simulink model "Siddarth_Kachu_FinalProject_Model"  (R2025a)
settings: Solver=FixedStepDiscrete  StartTime=0.0  StopTime=0.5  FixedStep=1e-6  RelTol=1e-3
model workspace (MAT data in the model file):
  AngularVelocity = Simulink.Parameter
  AngularVelocity.Value = 209.439510239
  AngularVelocity.Complexity = 'real'
  AngularVelocity.Dimensions = [1 1]
  AngularVelocity.DataType = 'auto'
  CounterTs = Simulink.Parameter
  CounterTs.Value = 20
  CounterTs.Complexity = 'real'
  CounterTs.Dimensions = [1 1]
  CounterTs.DataType = 'auto'
  Current_ZeroThreshold = Simulink.Parameter
  Current_ZeroThreshold.Value = 2.5
  Current_ZeroThreshold.Complexity = 'real'
  Current_ZeroThreshold.Dimensions = [1 1]
  Current_ZeroThreshold.DataType = 'auto'
  Nrpm = 2000
  OutputVoltages = [-5 -4 -3 -2 -1 0 1 2 3 4 5]
  RotorPoles = 8
  Rph = Simulink.Parameter
  Rph.Value = 0.4
  Rph.Complexity = 'real'
  Rph.Dimensions = [1 1]
  Rph.DataType = 'auto'
  Ts = Simulink.Parameter
  Ts.Value = 1e-06
  Ts.Complexity = 'real'
  Ts.Dimensions = [1 1]
  Ts.DataType = 'auto'
  Vdc = Simulink.Parameter
  Vdc.Value = 300
  Vdc.Complexity = 'real'
  Vdc.Dimensions = [1 1]
  Vdc.DataType = 'auto'
values from neighbouring files (symbols this model uses):
  elecAngleArray = [0 1.0000032 2.0000064 3.0000096 4.0000128 5.000016 6.0000192 7.0000224 8.0000256 9.0000288 10.000032 11.0000352 ... (360 elements, 360x1)]    [MPC_Controller_Final_Workspace.mat]
  LUT_currentMatrix = zeros(N_angles,N_fluxlink)    [Final_Project_Script.m]    (also in MPC_Controller_Final_Workspace.mat = [0 0 0 0 0 0 0 0 0 0 0 0 ... (129600 elements, 360x360)])
  targetArray = linspace(min(fluxLinkageMatrix(:)),max(fluxLinkageMatrix(:)),N_fluxlink)    [Final_Project_Script.m]    (also in MPC_Controller_Final_Workspace.mat = [0 0.00022373205571 0.000447464111421 0.000671196167131 0.00)
libraries: spsDiodeLib x12, spsIGBTDiodeLib x12, simulink x6, spsControlledCurrentSourceLib x3, spsVoltageMeasurementLib x3, spsDCVoltageSourceLib x2, simulink_need_slupdate x2, sps_lib x1
settings Model: Creator=kachus1  LastModifiedBy=kachus1
settings DataIOCC: ReturnWorkspaceOutputs=off

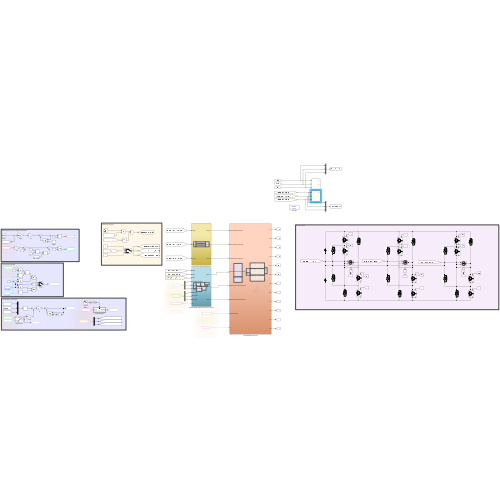
[thumbnail: Simulink's stored preview of the top-level diagram]
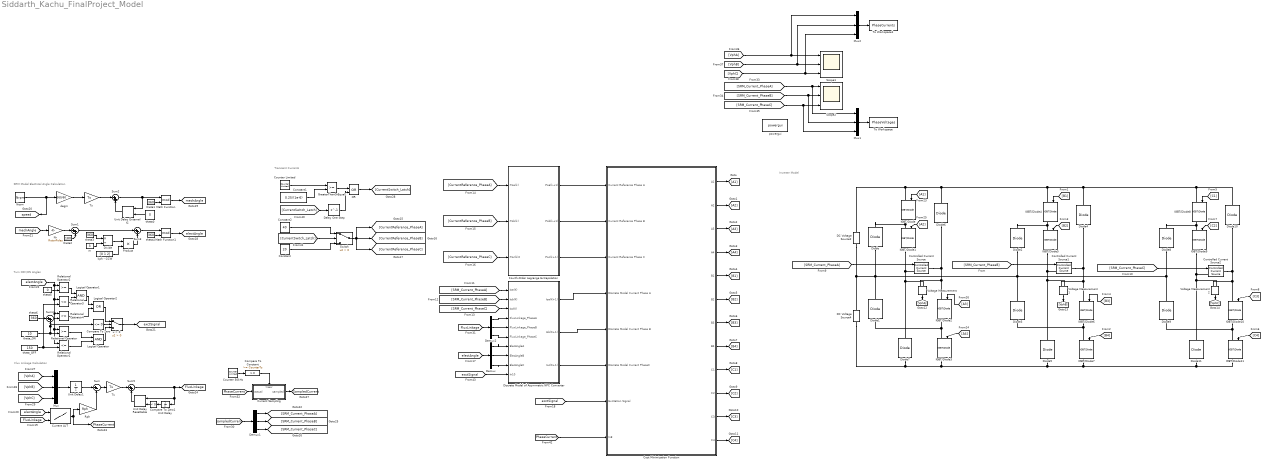
== system Siddarth_Kachu_FinalProject_Model ==
  note: Inverter Model
  note: Transient Currents
  note: Flux Linkage Calculation
  note: Turn OFF/ON Angles
  note: SRM Model Electrical Angle Calculation
  Compare To Constant : simulink/Logic and Bit Operations/Compare To Constant  relop=>=  const=CounterTs  OutDataTypeStr=boolean
  Compare To Zero : simulink/Logic and Bit Operations/Compare To Zero  relop=<=  OutDataTypeStr=boolean
  Compare To Zero1 : simulink/Logic and Bit Operations/Compare To Zero  relop=<  OutDataTypeStr=boolean
  Constant : Constant  Value=20
  Constant1 : Constant  Value=0.25/(1e-6)
  Constant2 : Constant  Value=40
  Controlled Current Source : spsControlledCurrentSourceLib/Controlled Current Source  Initialize=on  Source_Type=DC  Amplitude=0  Phase=0  Frequency=0  Measurements=None
  Controlled Current Source1 : spsControlledCurrentSourceLib/Controlled Current Source  Initialize=on  Source_Type=DC  Amplitude=0  Phase=0  Frequency=0  Measurements=None
  Controlled Current Source2 : spsControlledCurrentSourceLib/Controlled Current Source  Initialize=on  Source_Type=DC  Amplitude=0  Phase=0  Frequency=0  Measurements=None
  Cost Minimization Function : Subsystem
  Counter 50kHz : simulink/Sources/Counter Limited  uplimit=CounterTs  tsamp=-1
  Counter Limited : simulink/Sources/Counter Limited  uplimit=0.25/(1e-6)  tsamp=-1
  Current LUT : Lookup_n-D  BreakpointsForDimension1=elecAngleArray  BreakpointsForDimension2=targetArray  Table=LUT_currentMatrix  InternalRulePriority=Speed  RndMeth=Simplest
      settings: InputPortMap=u0,u1
  Current Sampling : Subsystem  TreatAsAtomicUnit=on
  DC Voltage Source2 : spsDCVoltageSourceLib/DC Voltage Source  Amplitude=150  Measurements=None
  DC Voltage Source4 : spsDCVoltageSourceLib/DC Voltage Source  Amplitude=150  Measurements=None
  Delay One Step : Delay  DelayLength=1
  Demux : Demux  Outputs=3
  Demux1 : Demux  Outputs=3
  Demux2 : Demux  Outputs=3
  Diode{,1..11} (12 alike) : spsDiodeLib/Diode  Ron=0.001  Lon=0  Vf=0  IC=0  UseSnubber=0  Rs=500  Cs=250e-9  Measurements=off
  Discrete Model of Asymmetric NPC Converter : Subsystem
  Divide : Product  Inputs=*/
  Fourth-Order Lagrange Extrapolation : Subsystem
  GreaterThanOrEqual : RelationalOperator  OutDataTypeStr=boolean  RndMeth=Simplest  InputSameDT=off
  IGBT/Diode{,1..11} (12 alike) : spsIGBTDiodeLib/IGBT//Diode  Ron=1e-3  Rs=1e5  Cs=inf  Measurements=on
  Logical Operator : Logic  AllPortsSameDT=off  OutDataTypeStr=boolean
  Logical Operator1 : Logic  AllPortsSameDT=off  OutDataTypeStr=boolean
  Logical Operator2 : Logic  Operator=OR  AllPortsSameDT=off  OutDataTypeStr=boolean
  Math Function : Math  Operator=mod  SignedPower=on
  Math Function1 : Math  Operator=mod  SignedPower=on
  Mux : Mux  Inputs=3
  Mux1 : Mux  Inputs=3
  Mux2 : Mux  Inputs=3
  Nr : Gain  Gain=RotorPoles
  Nrpm : Constant  Value=Nrpm
  OR : Logic  Operator=OR  IconShape=distinctive  AllPortsSameDT=off  OutDataTypeStr=boolean
  Product : Product
  Relational Operator : RelationalOperator  OutDataTypeStr=boolean  InputSameDT=off
  Relational Operator1 : RelationalOperator  Operator=<=  OutDataTypeStr=boolean  InputSameDT=off
  Relational Operator2 : RelationalOperator  OutDataTypeStr=boolean  InputSameDT=off
  Relational Operator3 : RelationalOperator  Operator=<=  OutDataTypeStr=boolean  InputSameDT=off
  Relational Operator4 : RelationalOperator  OutDataTypeStr=boolean  InputSameDT=off
  Rph : Gain  Gain=Rph
  Scope1 : Scope  NumInputPorts=3
      settings: ActiveDisplayYMinimum=-375.09564073144674  ActiveDisplayYMaximum=375.01062674793855
  Scope2 : Scope  NumInputPorts=3
      settings: ActiveDisplayYMinimum=-5.5949717067570885  ActiveDisplayYMaximum=48.44572805476993
  Sum : Sum  Inputs=|+-
  Sum{1..5} (5 alike) : Sum  Inputs=|++
  Switch : Switch  Criteria=u2 > Threshold  SaturateOnIntegerOverflow=off  InputSameDT=off
  To Workspace : ToWorkspace  VariableName=PhaseVoltages  SaveFormat=Structure With Time  SampleTime=-1
  To Workspace1 : ToWorkspace  VariableName=PhaseCurrents  SaveFormat=Structure With Time  SampleTime=-1
  Ts : Gain  Gain=Ts
  "Ts " : Gain  Gain=Ts
  Unit Delay : UnitDelay  SampleTime=-1  HasFrameUpgradeWarning=on
  Unit Delay External IC : simulink_need_slupdate/Unit Delay External IC  tsamp=-1
  Unit Delay Resettable : simulink_need_slupdate/Unit Delay Resettable  vinit=0.0  tsamp=-1
  Unit Delay1 : UnitDelay  SampleTime=-1  HasFrameUpgradeWarning=on
  Voltage Measurement : spsVoltageMeasurementLib/Voltage Measurement  PhasorSimulation=off  OutputType=Complex  PSBequivalent=0
  Voltage Measurement1 : spsVoltageMeasurementLib/Voltage Measurement  PhasorSimulation=off  OutputType=Complex  PSBequivalent=0
  Voltage Measurement2 : spsVoltageMeasurementLib/Voltage Measurement  PhasorSimulation=off  OutputType=Complex  PSBequivalent=0
  deg/s : Gain  Gain=360/60
  kph - CCW : Constant  Value=[0 1 2]
  m : Constant  Value=3
  powergui : sps_lib/powergui  Priority=1  SimulationMode=Discrete  SampleTime=1e-6  frequency=60  Iterations=50  frequencyindice=0  Pbase=100e6  ErrMax=1e-4  UnitsV=kV  UnitsW=MW  buscounter=0  FunctionMessages=off  echomessages=off  EnableUseOfTLC=off  CurrentSourceSwitches=off  DisableSnubberDevices=off  DisableRonSwitches=off  DisableVfSwitches=off  DisplayEquations=off  AutomaticDiscreteSolvers=off  SolverType=Tustin/Backward Euler (TBE)  Interpol=off  ExternalGateDelay=off  methode=off  Ts=100  x0status=blocks  SPID=on  SwTol=0  HookPort=off  NonlinearTolerance=1e-4  nMaxIteration=100  ContinueOnMaxIteration=off  RestoreLinks=warning  ResistiveCurrentMeasurement=off  Frange=[0:2:500]  Ylog=off  Xlog=on  ShowGrid=off  save=off  variable=ZData  structure=0  ZoomFFT=off  StartTime=0.0  cycles=1  DisplayStyle=1  fundamental=60  FreqAxis=off  MaxFrequency=1000  frequencyindicesteady=1  RmsSteady=1  display=off
  theta0 : Constant  Value=0
  theta{1,3..4,6} (4 alike) : Constant  Value=360
  theta2 : Constant  Value=180
  theta5 : Constant  Value=0
  theta_OFF : Constant  Value=150
  theta_ON : Constant  Value=10
  u > 0 : Switch  Criteria=u2 > Threshold  SaturateOnIntegerOverflow=off  InputSameDT=off
  tag scope: FluxLinkage=global, PhaseCurrent=global, SampledCurrent=global, electAngle=global, exctSignal=global, mechAngle=global, speed=global
  wires:
  [A2] -> IGBT/Diode1/1
  [A1] -> IGBT/Diode/1
  [A3] -> IGBT/Diode2/1
  [A4] -> IGBT/Diode3/1
  [B1] -> IGBT/Diode4/1
  [B2] -> IGBT/Diode5/1
  [B3] -> IGBT/Diode6/1
  [B4] -> IGBT/Diode7/1
  [C3] -> IGBT/Diode10/1
  [C4] -> IGBT/Diode11/1
  [C2] -> IGBT/Diode9/1
  [C1] -> IGBT/Diode8/1
  [SRM_Current_PhaseB] -> Controlled Current Source1/1
  [SRM_Current_PhaseA] -> Controlled Current Source/1
  [SRM_Current_PhaseC] -> Controlled Current Source2/1
  Cost Minimization Function/1(A1) -> [A1]
  Cost Minimization Function/2(A2) -> [A2]
  Cost Minimization Function/3(A3) -> [A3]
  Cost Minimization Function/4(A4) -> [A4]
  Cost Minimization Function/5(B1) -> [B1]
  Cost Minimization Function/6(B2) -> [B2]
  Cost Minimization Function/7(B3) -> [B3]
  Cost Minimization Function/8(B4) -> [B4]
  Cost Minimization Function/11(C3) -> [C3]
  Cost Minimization Function/10(C2) -> [C2]
  Cost Minimization Function/9(C1) -> [C1]
  Cost Minimization Function/12(C4) -> [C4]
  Discrete Model of Asymmetric NPC Converter/1(Ioa(K+1)) -> Cost Minimization Function/4(Discrete Model Current Phase A)
  Fourth-Order Lagrange Extrapolation/1(I*oa(k+1)) -> Cost Minimization Function/1(Current Reference Phase A)
  Fourth-Order Lagrange Extrapolation/2(I*ob(k+1)) -> Cost Minimization Function/2(Current Reference Phase B)
  Fourth-Order Lagrange Extrapolation/3(I*oc(k+1)) -> Cost Minimization Function/3(Current Reference Phase C)
  [SRM_Current_PhaseA] -> Discrete Model of Asymmetric NPC Converter/1(Ioa(K))
  [SRM_Current_PhaseB] -> Discrete Model of Asymmetric NPC Converter/2(Iob(K))
  [SRM_Current_PhaseC] -> Discrete Model of Asymmetric NPC Converter/3(Ioc(K))
  Voltage Measurement/1 -> [VphA]
  Voltage Measurement1/1 -> [VphB]
  Voltage Measurement2/1 -> [VphC]
  [CurrentReference_PhaseB] -> Fourth-Order Lagrange Extrapolation/2(I*ob(k))
  [CurrentReference_PhaseC] -> Fourth-Order Lagrange Extrapolation/3(I*oc(k)2)
  kph - CCW/1 -> Product/2
  Nrpm/1 -> [speed], deg/s/1
  "Ts "/1 -> Sum2/1
  Divide/1 -> Product/1
  deg/s/1 -> "Ts "/1
  theta0/1 -> Unit Delay External IC/2
  Nr/1 -> Sum1/1
  Math Function1/1 -> [electAngle]
  theta1/1 -> Math Function/2
  Product/1 -> Sum3/2
  m/1 -> Divide/2
  Sum3/1 -> Math Function1/1
  theta4/1 -> Math Function1/2
  [mechAngle] -> Nr/1
  Sum1/1 -> Sum3/1
  Math Function/1 -> [mechAngle]
  Sum2/1 -> Math Function/1, Unit Delay External IC/1
  theta3/1 -> Divide/1
  Unit Delay External IC/1 -> Sum2/2
  theta2/1 -> Sum1/2
  [electAngle] -> Demux/1
  Demux/1 -> Discrete Model of Asymmetric NPC Converter/7(ElecAngleA)
  Demux/2 -> Discrete Model of Asymmetric NPC Converter/8(ElecAngleB)
  Demux/3 -> Discrete Model of Asymmetric NPC Converter/9(ElecAngleC)
  Switch/1 -> [CurrentReference_PhaseA], [CurrentReference_PhaseC], [CurrentReference_PhaseB]
  theta6/1 -> Sum4/1
  theta5/1 -> Relational Operator2/2
  [electAngle] -> Relational Operator1/1, Relational Operator/1, Relational Operator4/1, Relational Operator3/1, Relational Operator2/1
  Relational Operator4/1 -> Logical Operator2/2
  Logical Operator1/1 -> Logical Operator2/1
  Relational Operator1/1 -> Logical Operator/2
  Relational Operator3/1 -> Logical Operator1/2
  theta_ON/1 -> Relational Operator/2, Compare To Zero/1, Sum4/2
  theta_OFF/1 -> Relational Operator3/2, Relational Operator1/2
  Logical Operator/1 -> u > 0/3
  Logical Operator2/1 -> u > 0/1
  Compare To Zero/1 -> u > 0/2
  Relational Operator/1 -> Logical Operator/1
  Sum4/1 -> Relational Operator4/2
  Relational Operator2/1 -> Logical Operator1/1
  u > 0/1 -> [exctSignal]
  [exctSignal] -> Cost Minimization Function/7(Excitation Signal)
  Discrete Model of Asymmetric NPC Converter/2(Iob(K+1)) -> Cost Minimization Function/5(Discrete Model Current Phase B)
  Discrete Model of Asymmetric NPC Converter/3(Ioc(K+1)) -> Cost Minimization Function/6(Discrete Model Current PhaseC)
  Unit Delay Resettable/1 -> Sum5/2
  Sum5/1 -> [FluxLinkage], Unit Delay/1, Unit Delay Resettable/1
  Current LUT/1 -> [PhaseCurrent], Rph/1
  Sum/1 -> Ts/1
  Rph/1 -> Sum/2
  Compare To Zero1/1 -> Unit Delay Resettable/2
  [FluxLinkage] -> Current LUT/2
  Unit Delay/1 -> Compare To Zero1/1
  [electAngle] -> Current LUT/1
  Ts/1 -> Sum5/1
  [VphB] -> Mux/2
  [VphC] -> Mux/3
  [VphA] -> Mux/1
  Mux/1 -> Unit Delay1/1
  [SampledCurrent] -> Demux1/1
  Demux1/1 -> [SRM_Current_PhaseA]
  Demux1/2 -> [SRM_Current_PhaseB]
  Demux1/3 -> [SRM_Current_PhaseC]
  [FluxLinkage] -> Demux2/1
  Demux2/1 -> Discrete Model of Asymmetric NPC Converter/4(FluxLinkage_PhaseA)
  Demux2/3 -> Discrete Model of Asymmetric NPC Converter/6(FluxLinkage_PhaseC)
  Demux2/2 -> Discrete Model of Asymmetric NPC Converter/5(FluxLinkage_PhaseB)
  [PhaseCurrent] -> Current Sampling/1(actual)
  Current Sampling/1(sampled) -> [SampledCurrent]
  Compare To Constant/1 -> Current Sampling/Trigger
  Counter 50kHz/1 -> Compare To Constant/1
  Unit Delay1/1 -> Sum/1
  [SRM_Current_PhaseC] -> Mux1/3, Scope2/3
  [SRM_Current_PhaseB] -> Mux1/2, Scope2/2
  [VphB] -> Mux2/2, Scope1/2
  [VphC] -> Mux2/3, Scope1/3
  Counter Limited/1 -> GreaterThanOrEqual/1
  Constant1/1 -> GreaterThanOrEqual/2
  Constant2/1 -> Switch/1
  Constant/1 -> Switch/3
  GreaterThanOrEqual/1 -> OR/1
  OR/1 -> [CurrentSwitch_Latch]
  [CurrentSwitch_Latch] -> Delay One Step/1
  Delay One Step/1 -> OR/2
  [CurrentSwitch_Latch] -> Switch/2
  [exctSignal] -> Discrete Model of Asymmetric NPC Converter/10(In10)
  [PhaseCurrent] -> Cost Minimization Function/8(In8)
  [CurrentReference_PhaseA] -> Fourth-Order Lagrange Extrapolation/1(I*oa(k))
  [SRM_Current_PhaseA] -> Mux1/1, Scope2/1
  Mux1/1 -> To Workspace/1
  [VphA] -> Mux2/1, Scope1/1
  Mux2/1 -> To Workspace1/1
  connections:
  Diode2/LConn1 -- Diode9/RConn1 -- Diode8/LConn1 -- Diode3/RConn1 -- DC Voltage Source4/RConn1 -- DC Voltage Source2/LConn1 -- Diode/LConn1 -- Diode1/RConn1
  Diode11/LConn1 -- IGBT/Diode11/RConn1 -- IGBT/Diode7/RConn1 -- Diode5/LConn1 -- Diode7/LConn1 -- DC Voltage Source4/LConn1 -- IGBT/Diode3/RConn1
  Diode10/RConn1 -- Diode4/RConn1 -- IGBT/Diode4/LConn1 -- Diode6/RConn1 -- DC Voltage Source2/RConn1 -- IGBT/Diode/LConn1 -- IGBT/Diode8/LConn1
  IGBT/Diode/RConn1 -- IGBT/Diode1/LConn1 -- Diode/RConn1
  IGBT/Diode3/LConn1 -- IGBT/Diode2/RConn1 -- Diode1/LConn1
  Diode6/LConn1 -- Voltage Measurement/LConn2 -- IGBT/Diode2/LConn1 -- Controlled Current Source/RConn1
  IGBT/Diode1/RConn1 -- Controlled Current Source/LConn1 -- Voltage Measurement/LConn1 -- Diode7/RConn1
  IGBT/Diode4/RConn1 -- IGBT/Diode5/LConn1 -- Diode2/RConn1
  Diode3/LConn1 -- IGBT/Diode7/LConn1 -- IGBT/Diode6/RConn1
  Diode4/LConn1 -- Controlled Current Source1/RConn1 -- Voltage Measurement1/LConn2 -- IGBT/Diode6/LConn1
  IGBT/Diode5/RConn1 -- Controlled Current Source1/LConn1 -- Voltage Measurement1/LConn1 -- Diode5/RConn1
  Diode9/LConn1 -- IGBT/Diode11/LConn1 -- IGBT/Diode10/RConn1
  IGBT/Diode8/RConn1 -- IGBT/Diode9/LConn1 -- Diode8/RConn1
  IGBT/Diode9/RConn1 -- Controlled Current Source2/LConn1 -- Voltage Measurement2/LConn1 -- Diode11/RConn1
  Diode10/LConn1 -- Controlled Current Source2/RConn1 -- Voltage Measurement2/LConn2 -- IGBT/Diode10/LConn1

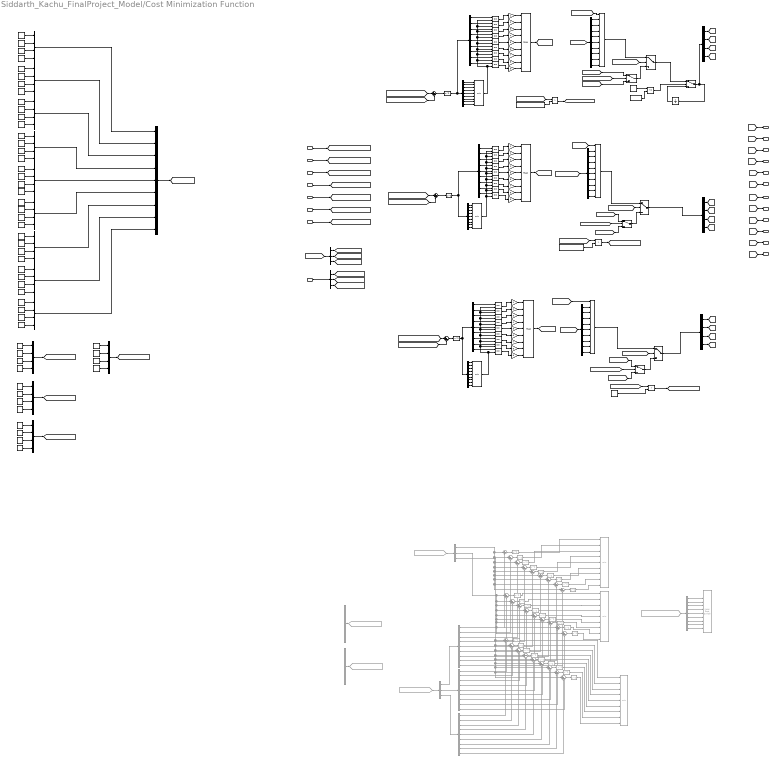
== system Siddarth_Kachu_FinalProject_Model/Cost Minimization Function ==
  note: ZeroVector_1
  note: Zero Vectors
  note: Excitation_Signal
  note: SwitchConfig
  note: Phase A
  note: Outputs
  note: Inputs
  note: Phase B
  note: Phase C
  Current Reference Phase A : Inport
  Current Reference Phase B : Inport  Port=2
  Current Reference Phase C : Inport  Port=3
  Discrete Model Current Phase A : Inport  Port=4
  Discrete Model Current Phase B : Inport  Port=5
  Discrete Model Current PhaseC : Inport  Port=6
  Excitation Signal : Inport  Port=7
  In8 : Inport  Port=8
  Constant : Constant  Value=Current_ZeroThreshold
  Constant{1..7,9..10,14..16,18..19,22,27..28,31,37,40,42..43,47..48} (24 alike) : Constant
  Constant{8,11..13,17,20..21,23..26,29..30,32..36,38..39,41,44..46,49..52} (28 alike) : Constant  Value=0
  Constant53 : Constant  Value=Current_ZeroThreshold
  Constant54 : Constant  Value=Current_ZeroThreshold
  Constant56 : Constant  Value=CounterTs
  Counter Limited : simulink/Sources/Counter Limited  uplimit=CounterTs  tsamp=-1
  Demux : Demux  Commented=on  Outputs=3
  Demux1 : Demux  Commented=on  Outputs=3
  Demux{6..8,10,13..15,18..19} (9 alike) : Demux  Outputs=9
  Demux11 : Demux
  Demux12 : Demux
  Demux16 : Demux
  Demux{2..5} (4 alike) : Demux  Commented=on  Outputs=9
  Demux22 : Demux  Outputs=3
  Demux9 : Demux  Outputs=3
  Equal{,1..26} (27 alike) : RelationalOperator  Operator===  OutDataTypeStr=boolean  RndMeth=Simplest  InputSameDT=off
  Equal28 : RelationalOperator  OutDataTypeStr=boolean  RndMeth=Simplest  InputSameDT=off
  From : From  Commented=on  GotoTag=NextStep_CurrentOutputs
  From1 : From  Commented=on  GotoTag=Reference_CurrentOutputs
  From9 : From  Commented=on  GotoTag=NextStep_CurrentOutputs_PhaseA
  Gain : Gain
  Gain1 : Gain  Gain=2
  Gain10 : Gain  Gain=2
  Gain11 : Gain  Gain=3
  Gain12 : Gain  Gain=4
  Gain13 : Gain  Gain=5
  Gain14 : Gain  Gain=6
  Gain15 : Gain  Gain=7
  Gain16 : Gain  Gain=8
  Gain17 : Gain  Gain=9
  Gain18 : Gain
  Gain19 : Gain  Gain=2
  Gain2 : Gain  Gain=3
  Gain20 : Gain  Gain=3
  Gain21 : Gain  Gain=4
  Gain22 : Gain  Gain=5
  Gain23 : Gain  Gain=6
  Gain24 : Gain  Gain=7
  Gain25 : Gain  Gain=8
  Gain26 : Gain  Gain=9
  Gain3 : Gain  Gain=4
  Gain4 : Gain  Gain=5
  Gain5 : Gain  Gain=6
  Gain6 : Gain  Gain=7
  Gain7 : Gain  Gain=8
  Gain8 : Gain  Gain=9
  Gain9 : Gain
  Goto2 : Goto  Commented=on  GotoTag=NextStep_CurrentOutputs
  Goto3 : Goto  Commented=on  GotoTag=Reference_CurrentOutputs
  GreaterThan : RelationalOperator  Operator=>  OutDataTypeStr=boolean  RndMeth=Simplest  InputSameDT=off
  GreaterThan1 : RelationalOperator  Operator=>  OutDataTypeStr=boolean  RndMeth=Simplest  InputSameDT=off
  GreaterThan2 : RelationalOperator  Operator=>  OutDataTypeStr=boolean  RndMeth=Simplest  InputSameDT=off
  Max : MinMax  Function=max  Inputs=9
  Max1 : MinMax  Function=max  Inputs=9
  Max2 : MinMax  Function=max  Inputs=9
  Min : MinMax  Commented=on  Inputs=9
  Min1 : MinMax  Commented=on  Inputs=9
  Min2 : MinMax  Inputs=9
  Min3 : MinMax  Commented=on  Inputs=9
  Min4 : MinMax  Inputs=9
  Min6 : MinMax  Inputs=9
  Multiport Switch : MultiPortSwitch  Commented=on  Inputs=9  SaturateOnIntegerOverflow=off  InputSameDT=off
  Multiport Switch1 : MultiPortSwitch  Inputs=9  DiagnosticForDefault=Warning  SaturateOnIntegerOverflow=off  InputSameDT=off
  Multiport Switch2 : MultiPortSwitch  Inputs=9  DiagnosticForDefault=Warning  SaturateOnIntegerOverflow=off  InputSameDT=off
  Multiport Switch3 : MultiPortSwitch  Inputs=9  DiagnosticForDefault=Warning  SaturateOnIntegerOverflow=off  InputSameDT=off
  Mux{,1,4..10,12..15} (13 alike) : Mux
  Mux11 : Mux  Inputs=9
  Mux2 : Mux  Commented=on  Inputs=3
  Mux3 : Mux  Commented=on  Inputs=3
  Square{,1..26} (27 alike) : Math  Commented=on  Operator=square
  Square27 : Math  Operator=square
  Square28 : Math  Operator=square
  Square30 : Math  Operator=square
  Sum{,1..26} (27 alike) : Sum  Commented=on  Inputs=|+-
  Sum27 : Sum  Inputs=|+-
  Sum28 : Sum  Inputs=|+-
  Sum29 : Sum  Inputs=|+-
  Switch{,1..6} (7 alike) : Switch  Criteria=u2 > Threshold  SaturateOnIntegerOverflow=off  InputSameDT=off
  Unit Delay : UnitDelay  SampleTime=-1  HasFrameUpgradeWarning=on
  A1 : Outport
  A2 : Outport  Port=2
  A3 : Outport  Port=3
  A4 : Outport  Port=4
  B1 : Outport  Port=5
  B2 : Outport  Port=6
  B3 : Outport  Port=7
  B4 : Outport  Port=8
  C1 : Outport  Port=9
  C2 : Outport  Port=10
  C3 : Outport  Port=11
  C4 : Outport  Port=12
  wires:
  Discrete Model Current Phase B/1 -> [NextStep_CurrentOutputs_PhaseB]
  Discrete Model Current Phase A/1 -> [NextStep_CurrentOutputs_PhaseA]
  Discrete Model Current PhaseC/1 -> [NextStep_CurrentOutputs_PhaseC]
  Current Reference Phase B/1 -> [Reference_CurrentOutputs_PhaseB]
  Current Reference Phase C/1 -> [Reference_CurrentOutputs_PhaseC]
  Current Reference Phase A/1 -> [Reference_CurrentOutputs_PhaseA]
  From1/1 -> Demux/1
  From/1 -> Demux1/1
  Demux1/1 -> Demux3/1
  Demux1/2 -> Demux2/1
  Demux1/3 -> Demux4/1
  Demux/1 -> Sum/1, Sum8/1, Sum7/1, Sum6/1, Sum5/1, Sum4/1, Sum3/1, Sum2/1, Sum1/1
  Demux3/1 -> Sum/2
  Demux3/2 -> Sum1/2
  Demux3/3 -> Sum2/2
  Demux3/4 -> Sum3/2
  Demux3/5 -> Sum4/2
  Demux3/6 -> Sum5/2
  Demux3/7 -> Sum6/2
  Demux3/8 -> Sum7/2
  Demux3/9 -> Sum8/2
  Sum/1 -> Square/1
  Sum1/1 -> Square1/1
  Sum2/1 -> Square2/1
  Sum3/1 -> Square3/1
  Sum4/1 -> Square4/1
  Sum5/1 -> Square5/1
  Sum6/1 -> Square6/1
  Sum7/1 -> Square7/1
  Sum8/1 -> Square8/1
  Demux/2 -> Sum9/1, Sum17/1, Sum16/1, Sum15/1, Sum14/1, Sum13/1, Sum12/1, Sum11/1, Sum10/1
  Sum14/1 -> Square14/1
  Sum9/1 -> Square9/1
  Sum11/1 -> Square11/1
  Sum15/1 -> Square15/1
  Sum16/1 -> Square16/1
  Demux2/9 -> Sum17/2
  Demux2/2 -> Sum10/2
  Demux2/5 -> Sum13/2
  Demux2/1 -> Sum9/2
  Demux2/8 -> Sum16/2
  Sum17/1 -> Square17/1
  Demux2/4 -> Sum12/2
  Demux2/3 -> Sum11/2
  Demux2/7 -> Sum15/2
  Sum12/1 -> Square12/1
  Sum10/1 -> Square10/1
  Sum13/1 -> Square13/1
  Demux2/6 -> Sum14/2
  Sum21/1 -> Square21/1
  Sum18/1 -> Square18/1
  Sum25/1 -> Square25/1
  Demux4/3 -> Sum19/2
  Demux4/8 -> Sum24/2
  Demux4/1 -> Sum26/2
  Demux4/9 -> Sum25/2
  Sum22/1 -> Square22/1
  Demux4/2 -> Sum18/2
  Sum19/1 -> Square19/1
  Sum26/1 -> Square26/1
  Sum24/1 -> Square24/1
  Sum23/1 -> Square23/1
  Sum20/1 -> Square20/1
  Demux/3 -> Sum26/1, Sum25/1, Sum24/1, Sum23/1, Sum22/1, Sum21/1, Sum20/1, Sum19/1, Sum18/1
  Demux4/5 -> Sum21/2
  Demux4/7 -> Sum23/2
  Demux4/4 -> Sum20/2
  Demux4/6 -> Sum22/2
  Square/1 -> Min/1
  Square1/1 -> Min/2
  Square2/1 -> Min/3
  Square3/1 -> Min/4
  Square4/1 -> Min/5
  Square5/1 -> Min/6
  Square6/1 -> Min/7
  Square7/1 -> Min/8
  Square8/1 -> Min/9
  Square9/1 -> Min1/1
  Square10/1 -> Min1/2
  Square11/1 -> Min1/3
  Square12/1 -> Min1/4
  Square13/1 -> Min1/5
  Square14/1 -> Min1/6
  Square15/1 -> Min1/7
  Square16/1 -> Min1/8
  Square17/1 -> Min1/9
  Square26/1 -> Min3/1
  Square18/1 -> Min3/2
  Square19/1 -> Min3/3
  Square20/1 -> Min3/4
  Square21/1 -> Min3/5
  Square22/1 -> Min3/6
  Square23/1 -> Min3/7
  Square24/1 -> Min3/8
  Square25/1 -> Min3/9
  Sum27/1 -> Square27/1
  Sum28/1 -> Square28/1
  Sum29/1 -> Square30/1
  Square28/1 -> Demux8/1, Demux14/1
  ? -> Mux2/2
  ? -> Mux3/3
  Mux2/1 -> Goto2/1
  Mux3/1 -> Goto3/1
  ? -> Mux3/2
  ? -> Mux2/3
  ? -> Mux3/1
  ? -> Mux2/1
  [NextStep_CurrentOutputs_PhaseA] -> Sum27/2
  [Reference_CurrentOutputs_PhaseB] -> Sum28/1
  [NextStep_CurrentOutputs_PhaseB] -> Sum28/2
  [NextStep_CurrentOutputs_PhaseC] -> Sum29/2
  [Reference_CurrentOutputs_PhaseC] -> Sum29/1
  Demux7/1 -> Min2/1
  Demux7/2 -> Min2/2
  Demux7/3 -> Min2/3
  Demux7/4 -> Min2/4
  Demux7/5 -> Min2/5
  Demux7/6 -> Min2/6
  Demux7/7 -> Min2/7
  Demux7/8 -> Min2/8
  Demux7/9 -> Min2/9
  Demux8/1 -> Min4/1
  Demux8/2 -> Min4/2
  Demux8/3 -> Min4/3
  Demux8/4 -> Min4/4
  Demux8/5 -> Min4/5
  Demux8/6 -> Min4/6
  Demux8/7 -> Min4/7
  Demux8/8 -> Min4/8
  Demux8/9 -> Min4/9
  Demux5/9 -> Multiport Switch/10
  Demux5/3 -> Multiport Switch/4
  From9/1 -> Demux5/1
  Demux5/1 -> Multiport Switch/2
  Demux5/4 -> Multiport Switch/5
  Demux5/8 -> Multiport Switch/9
  Demux5/7 -> Multiport Switch/8
  Demux5/6 -> Multiport Switch/7
  Demux5/5 -> Multiport Switch/6
  Demux5/2 -> Multiport Switch/3
  Constant1/1 -> Mux/1
  Constant2/1 -> Mux/2
  Constant3/1 -> Mux/3
  Constant4/1 -> Mux/4
  Constant8/1 -> Mux1/4
  Constant7/1 -> Mux1/3
  Constant6/1 -> Mux1/2
  Constant5/1 -> Mux1/1
  Constant10/1 -> Mux4/2
  Constant12/1 -> Mux4/4
  Constant9/1 -> Mux4/1
  Constant11/1 -> Mux4/3
  Constant14/1 -> Mux5/2
  Constant16/1 -> Mux5/4
  Constant13/1 -> Mux5/1
  Constant15/1 -> Mux5/3
  Constant19/1 -> Mux6/3
  Constant20/1 -> Mux6/4
  Constant18/1 -> Mux6/2
  Constant17/1 -> Mux6/1
  Constant21/1 -> Mux7/1
  Constant24/1 -> Mux7/4
  Constant23/1 -> Mux7/3
  Constant22/1 -> Mux7/2
  Constant27/1 -> Mux8/3
  Constant28/1 -> Mux8/4
  Constant26/1 -> Mux8/2
  Constant25/1 -> Mux8/1
  Constant29/1 -> Mux9/1
  Constant32/1 -> Mux9/4
  Constant34/1 -> Mux10/2
  Constant30/1 -> Mux9/2
  Constant33/1 -> Mux10/1
  Constant31/1 -> Mux9/3
  Constant36/1 -> Mux10/4
  Constant35/1 -> Mux10/3
  Mux/1 -> Mux11/1
  Mux1/1 -> Mux11/2
  Mux4/1 -> Mux11/3
  Mux5/1 -> Mux11/4
  Mux6/1 -> Mux11/5
  Mux7/1 -> Mux11/6
  Mux8/1 -> Mux11/7
  Mux9/1 -> Mux11/8
  Mux10/1 -> Mux11/9
  Mux11/1 -> [Switch_Configs]
  Square27/1 -> Demux7/1, Demux10/1
  Demux6/1 -> Multiport Switch1/2
  Demux6/2 -> Multiport Switch1/3
  Demux6/3 -> Multiport Switch1/4
  Demux6/4 -> Multiport Switch1/5
  Demux6/5 -> Multiport Switch1/6
  Demux6/6 -> Multiport Switch1/7
  Demux6/7 -> Multiport Switch1/8
  Demux6/8 -> Multiport Switch1/9
  Demux6/9 -> Multiport Switch1/10
  [Switch_Configs] -> Demux6/1
  Demux10/1 -> Equal/1
  Min2/1 -> Equal6/2, Equal5/2, Equal/2, Equal1/2, Equal2/2, Equal3/2, Equal4/2, Equal7/2, Equal8/2
  Demux10/2 -> Equal1/1
  Demux10/3 -> Equal2/1
  Demux10/4 -> Equal3/1
  Demux10/5 -> Equal4/1
  Demux10/6 -> Equal5/1
  Demux10/7 -> Equal6/1
  Demux10/8 -> Equal7/1
  Demux10/9 -> Equal8/1
  Equal/1 -> Gain/1
  Equal1/1 -> Gain1/1
  Equal3/1 -> Gain3/1
  Equal4/1 -> Gain4/1
  Equal5/1 -> Gain5/1
  Equal6/1 -> Gain6/1
  Equal7/1 -> Gain7/1
  Equal8/1 -> Gain8/1
  Gain/1 -> Max/1
  Gain1/1 -> Max/2
  Gain2/1 -> Max/3
  Equal2/1 -> Gain2/1
  Gain3/1 -> Max/4
  Gain4/1 -> Max/5
  Gain5/1 -> Max/6
  Gain6/1 -> Max/7
  Gain7/1 -> Max/8
  Gain8/1 -> Max/9
  Demux11/1 -> [A1]
  Demux11/2 -> [A2]
  Demux11/3 -> [A3]
  Demux11/4 -> [A4]
  [A1] -> A1/1
  [A2] -> A2/1
  [A3] -> A3/1
  [A4] -> A4/1
  Equal10/1 -> Gain10/1
  Equal9/1 -> Gain9/1
  Demux12/2 -> [B2]
  Demux12/3 -> [B3]
  Demux12/1 -> [B1]
  Demux12/4 -> [B4]
  Gain12/1 -> Max1/4
  Gain17/1 -> Max1/9
  Equal16/1 -> Gain16/1
  Gain10/1 -> Max1/2
  Gain13/1 -> Max1/5
  Equal13/1 -> Gain13/1
  Equal15/1 -> Gain15/1
  Gain14/1 -> Max1/6
  [Switch_Configs] -> Demux13/1
  Gain11/1 -> Max1/3
  Equal17/1 -> Gain17/1
  Demux13/3 -> Multiport Switch2/4
  Gain9/1 -> Max1/1
  Gain16/1 -> Max1/8
  Demux13/9 -> Multiport Switch2/10
  Demux13/8 -> Multiport Switch2/9
  Demux13/7 -> Multiport Switch2/8
  Demux13/4 -> Multiport Switch2/5
  Equal11/1 -> Gain11/1
  Demux13/1 -> Multiport Switch2/2
  Equal12/1 -> Gain12/1
  Demux13/6 -> Multiport Switch2/7
  Gain15/1 -> Max1/7
  Demux13/5 -> Multiport Switch2/6
  Demux13/2 -> Multiport Switch2/3
  Equal14/1 -> Gain14/1
  Min4/1 -> Equal9/2, Equal10/2, Equal11/2, Equal12/2, Equal13/2, Equal14/2, Equal15/2, Equal16/2, Equal17/2
  Demux14/1 -> Equal9/1
  Demux14/2 -> Equal10/1
  Demux14/3 -> Equal11/1
  Demux14/4 -> Equal12/1
  Demux14/5 -> Equal13/1
  Demux14/6 -> Equal14/1
  Demux14/7 -> Equal15/1
  Demux14/8 -> Equal16/1
  Demux14/9 -> Equal17/1
  [B1] -> B1/1
  [B2] -> B2/1
  [B3] -> B3/1
  [B4] -> B4/1
  Demux16/2 -> [C2]
  Demux15/1 -> Equal18/1
  Demux15/7 -> Equal24/1
  Demux15/8 -> Equal25/1
  Equal19/1 -> Gain19/1
  Equal18/1 -> Gain18/1
  Demux16/1 -> [C1]
  Demux15/3 -> Equal20/1
  Demux15/4 -> Equal21/1
  Demux15/5 -> Equal22/1
  Min6/1 -> Equal24/2, Equal23/2, Equal18/2, Equal19/2, Equal20/2, Equal21/2, Equal22/2, Equal25/2, Equal26/2
  Gain21/1 -> Max2/4
  Demux15/6 -> Equal23/1
  Equal25/1 -> Gain25/1
  Demux15/9 -> Equal26/1
  Gain19/1 -> Max2/2
  Gain22/1 -> Max2/5
  Equal22/1 -> Gain22/1
  Gain20/1 -> Max2/3
  [Switch_Configs] -> Demux18/1
  Equal26/1 -> Gain26/1
  Demux18/3 -> Multiport Switch3/4
  Gain18/1 -> Max2/1
  Gain25/1 -> Max2/8
  Demux18/2 -> Multiport Switch3/3
  Equal23/1 -> Gain23/1
  Demux18/4 -> Multiport Switch3/5
  Equal20/1 -> Gain20/1
  Demux18/8 -> Multiport Switch3/9
  Demux18/9 -> Multiport Switch3/10
  Demux18/1 -> Multiport Switch3/2
  Equal21/1 -> Gain21/1
  Demux18/6 -> Multiport Switch3/7
  Gain24/1 -> Max2/7
  Equal24/1 -> Gain24/1
  Gain23/1 -> Max2/6
  Demux19/6 -> Min6/6
  Demux19/2 -> Min6/2
  Demux16/4 -> [C4]
  Demux19/8 -> Min6/8
  Gain26/1 -> Max2/9
  Square30/1 -> Demux19/1, Demux15/1
  Demux16/3 -> [C3]
  Demux19/7 -> Min6/7
  Demux15/2 -> Equal19/1
  Demux19/4 -> Min6/4
  Demux19/3 -> Min6/3
  Demux18/5 -> Multiport Switch3/6
  Demux19/1 -> Min6/1
  Demux19/5 -> Min6/5
  Demux18/7 -> Multiport Switch3/8
  [C1] -> C1/1
  [C2] -> C2/1
  [C3] -> C3/1
  [C4] -> C4/1
  Demux19/9 -> Min6/9
  Excitation Signal/1 -> [Excitation_Signal]
  Demux9/1 -> [Excitation_Signal_A]
  Demux9/2 -> [Excitation_Signal_B]
  Demux9/3 -> [Excitation_Signal_C]
  [Excitation_Signal] -> Demux9/1
  Constant38/1 -> Mux12/3
  Constant40/1 -> Mux12/1
  Constant39/1 -> Mux12/4
  Constant37/1 -> Mux12/2
  Constant43/1 -> Mux13/3
  Constant42/1 -> Mux13/2
  Constant44/1 -> Mux13/4
  Constant41/1 -> Mux13/1
  Constant46/1 -> Mux14/2
  Constant45/1 -> Mux14/1
  Constant48/1 -> Mux14/4
  Constant47/1 -> Mux14/3
  Mux12/1 -> [ZeroVector_1]
  Mux13/1 -> [ZeroVector_2]
  Mux14/1 -> [ZeroVector_3]
  [Excitation_Signal_A] -> Switch/2
  Switch3/1 -> Switch/3
  Switch4/1 -> Switch1/3
  [Excitation_Signal_B] -> Switch1/2
  Multiport Switch2/1 -> Switch1/1
  Switch1/1 -> Demux12/1
  [Excitation_Signal_C] -> Switch2/2
  Multiport Switch3/1 -> Switch2/1
  Switch2/1 -> Demux16/1
  Constant50/1 -> Mux15/2
  Constant51/1 -> Mux15/3
  Constant49/1 -> Mux15/1
  Constant52/1 -> Mux15/4
  Mux15/1 -> [NegativeVector]
  [Current_Condition_PhaseA] -> Switch3/2
  [NegativeVector] -> Switch3/1
  [ZeroVector_1] -> Switch3/3
  Max/1 -> [Index_Vector_A]
  [Index_Vector_A] -> Multiport Switch1/1
  Max1/1 -> [Index_Vector_B]
  [Index_Vector_B] -> Multiport Switch2/1
  [ZeroVector_1] -> Switch4/3
  [NegativeVector] -> Switch4/1
  [Current_Condition_PhaseB] -> Switch4/2
  Max2/1 -> [Index_Vector_C]
  [Index_Vector_C] -> Multiport Switch3/1
  Switch5/1 -> Switch2/3
  [Current_Condition_PhaseC] -> Switch5/2
  [ZeroVector_1] -> Switch5/3
  [NegativeVector] -> Switch5/1
  [Sample_CurrentPhaseA] -> GreaterThan/1
  Constant/1 -> GreaterThan/2
  GreaterThan/1 -> [Current_Condition_PhaseA]
  Constant53/1 -> GreaterThan1/2
  GreaterThan1/1 -> [Current_Condition_PhaseB]
  [Sample_CurrentPhaseB] -> GreaterThan1/1
  [Sample_CurrentPhaseC] -> GreaterThan2/1
  Constant54/1 -> GreaterThan2/2
  GreaterThan2/1 -> [Current_Condition_PhaseC]
  Demux22/3 -> [Sample_CurrentPhaseC]
  Demux22/1 -> [Sample_CurrentPhaseA]
  Demux22/2 -> [Sample_CurrentPhaseB]
  In8/1 -> Demux22/1
  Switch6/1 -> Demux11/1, Unit Delay/1
  Unit Delay/1 -> Switch6/3
  Counter Limited/1 -> Equal28/1
  Constant56/1 -> Equal28/2
  Equal28/1 -> Switch6/2
  [Reference_CurrentOutputs_PhaseA] -> Sum27/1
  Multiport Switch1/1 -> Switch/1
  Switch/1 -> Switch6/1

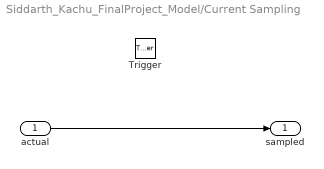
== system Siddarth_Kachu_FinalProject_Model/Current Sampling ==
  actual : Inport
  Trigger : TriggerPort  VariantControl=Variant
  sampled : Outport
  wires:
  actual/1 -> sampled/1

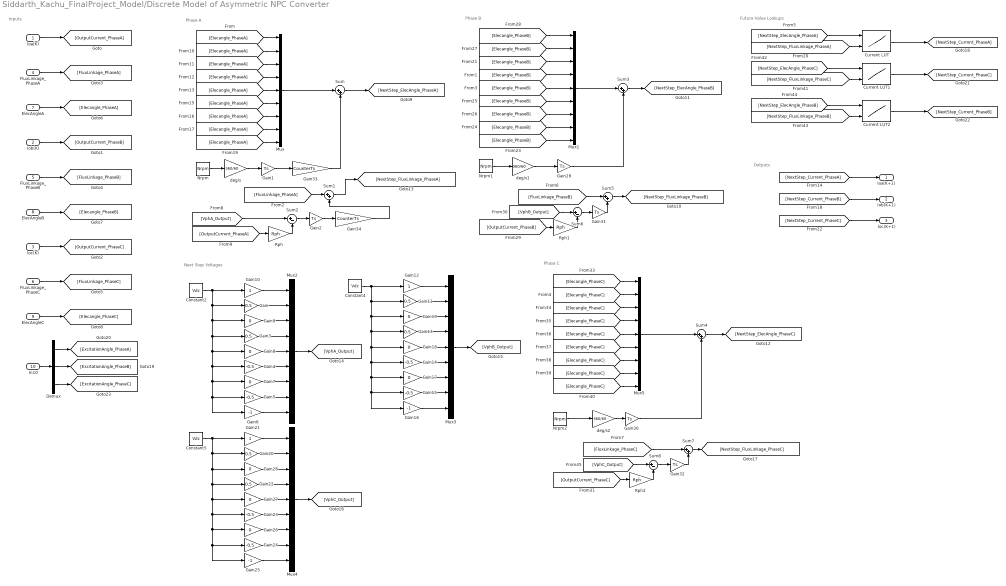
== system Siddarth_Kachu_FinalProject_Model/Discrete Model of Asymmetric NPC Converter ==
  note: Phase C
  note: Phase B
  note: Phase A
  note: Next Step Voltages
  note: Outputs
  note: Inputs
  note: Future Value Lookups
  Ioa(K) : Inport
  Iob(K) : Inport  Port=2
  Ioc(K) : Inport  Port=3
  FluxLinkage_PhaseA : Inport  Port=4
  FluxLinkage_PhaseB : Inport  Port=5
  FluxLinkage_PhaseC : Inport  Port=6
  ElecAngleA : Inport  Port=7
  ElecAngleB : Inport  Port=8
  ElecAngleC : Inport  Port=9
  In10 : Inport  Port=10
  Constant2 : Constant  Value=Vdc
  Constant4 : Constant  Value=Vdc
  Constant5 : Constant  Value=Vdc
  Current LUT : Lookup_n-D  BreakpointsForDimension1=elecAngleArray  BreakpointsForDimension2=targetArray  Table=LUT_currentMatrix  InternalRulePriority=Speed  RndMeth=Simplest
      settings: InputPortMap=u0,u1
  Current LUT1 : Lookup_n-D  BreakpointsForDimension1=elecAngleArray  BreakpointsForDimension2=targetArray  Table=LUT_currentMatrix  InternalRulePriority=Speed  RndMeth=Simplest
      settings: InputPortMap=u0,u1
  Current LUT2 : Lookup_n-D  BreakpointsForDimension1=elecAngleArray  BreakpointsForDimension2=targetArray  Table=LUT_currentMatrix  InternalRulePriority=Speed  RndMeth=Simplest
      settings: InputPortMap=u0,u1
  Demux : Demux  Outputs=3
  Gain{,3,11,13,20,22} (6 alike) : Gain  Gain=0.5
  Gain{1..2,29..32} (6 alike) : Gain  Gain=Ts
  Gain10 : Gain
  Gain12 : Gain
  Gain{4..5,14..15,23..24} (6 alike) : Gain  Gain=-0.5
  Gain16 : Gain  Gain=-1
  Gain{7..9,17..19,26..28} (9 alike) : Gain  Gain=0
  Gain21 : Gain
  Gain25 : Gain  Gain=-1
  Gain33 : Gain  Gain=CounterTs
  Gain34 : Gain  Gain=CounterTs
  Gain6 : Gain  Gain=-1
  Mux{,1..5} (6 alike) : Mux  Inputs=9
  Nrpm : Constant  Value=Nrpm
  Nrpm1 : Constant  Value=Nrpm
  Nrpm2 : Constant  Value=Nrpm
  Rph : Gain  Gain=Rph
  Rph1 : Gain  Gain=Rph
  Rph2 : Gain  Gain=Rph
  Sum{,1,3..5,7} (6 alike) : Sum  Inputs=|++
  Sum2 : Sum  Inputs=|+-
  Sum6 : Sum  Inputs=|+-
  Sum8 : Sum  Inputs=|+-
  deg/s : Gain  Gain=360/60
  deg/s1 : Gain  Gain=360/60
  deg/s2 : Gain  Gain=360/60
  Ioa(K+1) : Outport
  Iob(K+1) : Outport  Port=2
  Ioc(K+1) : Outport  Port=3
  wires:
  Ioa(K)/1 -> [OutputCurrent_PhaseA]
  Iob(K)/1 -> [OutputCurrent_PhaseB]
  Ioc(K)/1 -> [OutputCurrent_PhaseC]
  FluxLinkage_PhaseA/1 -> [FluxLinkage_PhaseA]
  FluxLinkage_PhaseB/1 -> [FluxLinkage_PhaseB]
  FluxLinkage_PhaseC/1 -> [FluxLinkage_PhaseC]
  ElecAngleA/1 -> [Elecangle_PhaseA]
  ElecAngleB/1 -> [Elecangle_PhaseB]
  ElecAngleC/1 -> [Elecangle_PhaseC]
  Constant2/1 -> Gain/1, Gain9/1, Gain3/1, Gain8/1, Gain4/1, Gain7/1, Gain5/1, Gain6/1, Gain10/1
  Gain/1 -> Mux2/2
  Gain3/1 -> Mux2/4
  Gain4/1 -> Mux2/6
  Gain5/1 -> Mux2/8
  Gain6/1 -> Mux2/9
  Gain7/1 -> Mux2/7
  Gain8/1 -> Mux2/5
  Gain9/1 -> Mux2/3
  Gain10/1 -> Mux2/1
  Mux2/1 -> [VphA_Output]
  Gain17/1 -> Mux3/7
  Gain12/1 -> Mux3/1
  Gain11/1 -> Mux3/2
  Gain19/1 -> Mux3/3
  Gain13/1 -> Mux3/4
  Gain18/1 -> Mux3/5
  Constant4/1 -> Gain11/1, Gain19/1, Gain13/1, Gain18/1, Gain14/1, Gain17/1, Gain15/1, Gain16/1, Gain12/1
  Gain16/1 -> Mux3/9
  Gain15/1 -> Mux3/8
  Gain14/1 -> Mux3/6
  Mux3/1 -> [VphB_Output]
  Gain26/1 -> Mux4/7
  Gain21/1 -> Mux4/1
  Gain20/1 -> Mux4/2
  Gain28/1 -> Mux4/3
  Gain22/1 -> Mux4/4
  Gain27/1 -> Mux4/5
  Constant5/1 -> Gain20/1, Gain28/1, Gain22/1, Gain27/1, Gain23/1, Gain26/1, Gain24/1, Gain25/1, Gain21/1
  Gain25/1 -> Mux4/9
  Gain24/1 -> Mux4/8
  Gain23/1 -> Mux4/6
  Mux4/1 -> [VphC_Output]
  [NextStep_Current_PhaseB] -> Iob(K+1)/1
  [NextStep_Current_PhaseC] -> Ioc(K+1)/1
  Current LUT/1 -> [NextStep_Current_PhaseA]
  [NextStep_ElecAngle_PhaseA] -> Current LUT/1
  [NextStep_FluxLinkage_PhaseA] -> Current LUT/2
  deg/s/1 -> Gain1/1
  Nrpm/1 -> deg/s/1
  Sum/1 -> [NextStep_ElecAngle_PhaseA]
  [FluxLinkage_PhaseA] -> Sum1/1
  [VphA_Output] -> Sum2/1
  Sum2/1 -> Gain2/1
  Rph/1 -> Sum2/2
  [OutputCurrent_PhaseA] -> Rph/1
  Sum3/1 -> [NextStep_ElecAngle_PhaseB]
  Nrpm1/1 -> deg/s1/1
  deg/s1/1 -> Gain29/1
  Mux5/1 -> Sum4/1
  Sum4/1 -> [NextStep_ElecAngle_PhaseC]
  Nrpm2/1 -> deg/s2/1
  deg/s2/1 -> Gain30/1
  Sum1/1 -> [NextStep_FluxLinkage_PhaseA]
  [Elecangle_PhaseA] -> Mux/1
  [Elecangle_PhaseA] -> Mux/2
  [Elecangle_PhaseA] -> Mux/5
  [Elecangle_PhaseA] -> Mux/4
  [Elecangle_PhaseA] -> Mux/3
  [Elecangle_PhaseA] -> Mux/6
  [Elecangle_PhaseA] -> Mux/7
  [Elecangle_PhaseA] -> Mux/8
  [Elecangle_PhaseA] -> Mux/9
  Mux/1 -> Sum/1
  [Elecangle_PhaseB] -> Mux1/5
  [Elecangle_PhaseB] -> Mux1/1
  [Elecangle_PhaseB] -> Mux1/2
  [Elecangle_PhaseB] -> Mux1/3
  [Elecangle_PhaseB] -> Mux1/4
  [Elecangle_PhaseB] -> Mux1/6
  [Elecangle_PhaseB] -> Mux1/7
  [Elecangle_PhaseB] -> Mux1/8
  [Elecangle_PhaseB] -> Mux1/9
  Mux1/1 -> Sum3/1
  Sum5/1 -> [NextStep_FluxLinkage_PhaseB]
  Sum6/1 -> Gain31/1
  [FluxLinkage_PhaseB] -> Sum5/1
  [OutputCurrent_PhaseB] -> Rph1/1
  Gain31/1 -> Sum5/2
  [VphB_Output] -> Sum6/1
  Rph1/1 -> Sum6/2
  Sum8/1 -> Gain32/1
  [VphC_Output] -> Sum8/1
  Gain32/1 -> Sum7/2
  [OutputCurrent_PhaseC] -> Rph2/1
  Sum7/1 -> [NextStep_FluxLinkage_PhaseC]
  [FluxLinkage_PhaseC] -> Sum7/1
  Rph2/1 -> Sum8/2
  [Elecangle_PhaseC] -> Mux5/1
  [Elecangle_PhaseC] -> Mux5/9
  [Elecangle_PhaseC] -> Mux5/8
  [Elecangle_PhaseC] -> Mux5/7
  [Elecangle_PhaseC] -> Mux5/6
  [Elecangle_PhaseC] -> Mux5/5
  [Elecangle_PhaseC] -> Mux5/4
  [Elecangle_PhaseC] -> Mux5/3
  [Elecangle_PhaseC] -> Mux5/2
  Current LUT1/1 -> [NextStep_Current_PhaseC]
  [NextStep_ElecAngle_PhaseC] -> Current LUT1/1
  [NextStep_FluxLinkage_PhaseC] -> Current LUT1/2
  [NextStep_FluxLinkage_PhaseB] -> Current LUT2/2
  Current LUT2/1 -> [NextStep_Current_PhaseB]
  [NextStep_ElecAngle_PhaseB] -> Current LUT2/1
  Gain1/1 -> Gain33/1
  Gain33/1 -> Sum/2
  Gain29/1 -> Sum3/2
  Gain30/1 -> Sum4/2
  Gain2/1 -> Gain34/1
  Gain34/1 -> Sum1/2
  In10/1 -> Demux/1
  Demux/2 -> [ExcitationAngle_PhaseB]
  Demux/1 -> [ExcitationAngle_PhaseA]
  Demux/3 -> [ExcitationAngle_PhaseC]
  [NextStep_Current_PhaseA] -> Ioa(K+1)/1

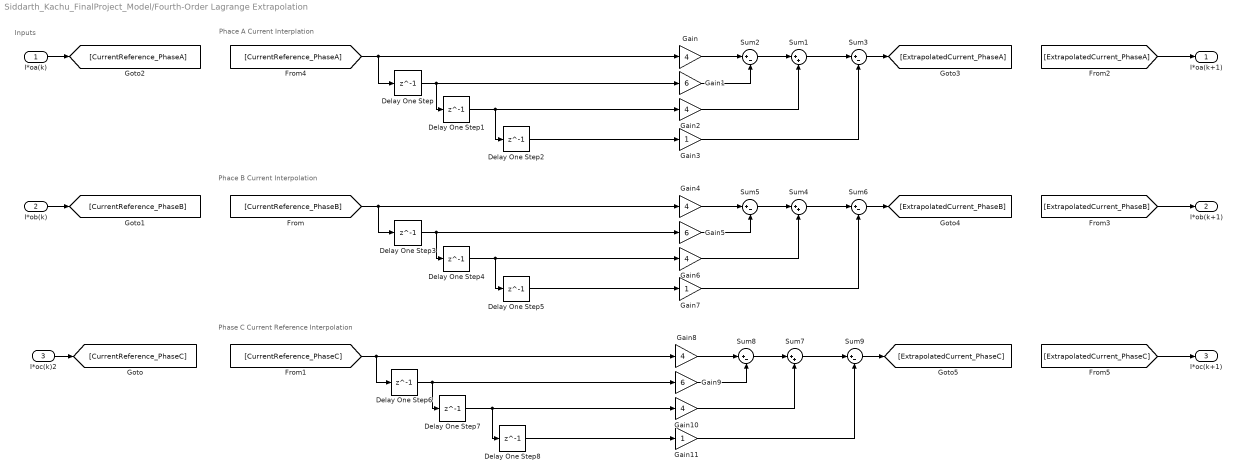
== system Siddarth_Kachu_FinalProject_Model/Fourth-Order Lagrange Extrapolation ==
  note: Inputs
  note: Phace A Current Interplation
  note: Phace B Current Interpolation
  note: Phase C Current Reference Interpolation
  I*oa(k) : Inport
  I*ob(k) : Inport  Port=2
  I*oc(k)2 : Inport  Port=3
  Delay One Step{,1..8} (9 alike) : Delay  DelayLength=1
  Gain{,2,4,6,8,10} (6 alike) : Gain  Gain=4
  Gain1 : Gain  Gain=6
  Gain11 : Gain
  Gain3 : Gain
  Gain5 : Gain  Gain=6
  Gain7 : Gain
  Gain9 : Gain  Gain=6
  Sum1 : Sum  Inputs=|++
  Sum{2..3,5..6,8..9} (6 alike) : Sum  Inputs=|+-
  Sum4 : Sum  Inputs=|++
  Sum7 : Sum  Inputs=|++
  I*oa(k+1) : Outport
  I*ob(k+1) : Outport  Port=2
  I*oc(k+1) : Outport  Port=3
  wires:
  Gain/1 -> Sum2/1
  Delay One Step/1 -> Delay One Step1/1, Gain1/1
  Gain1/1 -> Sum2/2
  Sum2/1 -> Sum1/1
  Gain2/1 -> Sum1/2
  Gain3/1 -> Sum3/2
  Delay One Step1/1 -> Delay One Step2/1, Gain2/1
  Delay One Step2/1 -> Gain3/1
  Sum1/1 -> Sum3/1
  Gain4/1 -> Sum5/1
  Sum5/1 -> Sum4/1
  Gain5/1 -> Sum5/2
  Sum4/1 -> Sum6/1
  Gain7/1 -> Sum6/2
  Delay One Step4/1 -> Delay One Step5/1, Gain6/1
  Delay One Step5/1 -> Gain7/1
  Gain6/1 -> Sum4/2
  Delay One Step3/1 -> Delay One Step4/1, Gain5/1
  Gain8/1 -> Sum8/1
  Sum8/1 -> Sum7/1
  Gain9/1 -> Sum8/2
  Sum7/1 -> Sum9/1
  Gain11/1 -> Sum9/2
  Delay One Step7/1 -> Delay One Step8/1, Gain10/1
  Delay One Step8/1 -> Gain11/1
  Gain10/1 -> Sum7/2
  Delay One Step6/1 -> Delay One Step7/1, Gain9/1
  I*oc(k)2/1 -> [CurrentReference_PhaseC]
  [CurrentReference_PhaseC] -> Gain8/1, Delay One Step6/1
  I*ob(k)/1 -> [CurrentReference_PhaseB]
  [CurrentReference_PhaseB] -> Gain4/1, Delay One Step3/1
  I*oa(k)/1 -> [CurrentReference_PhaseA]
  [CurrentReference_PhaseA] -> Gain/1, Delay One Step/1
  Sum3/1 -> [ExtrapolatedCurrent_PhaseA]
  [ExtrapolatedCurrent_PhaseA] -> I*oa(k+1)/1
  Sum6/1 -> [ExtrapolatedCurrent_PhaseB]
  [ExtrapolatedCurrent_PhaseB] -> I*ob(k+1)/1
  Sum9/1 -> [ExtrapolatedCurrent_PhaseC]
  [ExtrapolatedCurrent_PhaseC] -> I*oc(k+1)/1
